simulink model "sample2"  (R2017b)
settings: Solver=VariableStepAuto  StartTime=0.0  StopTime=10.0  RelTol=1e-3
settings Model: Creator=aki  LastModifiedBy=aki

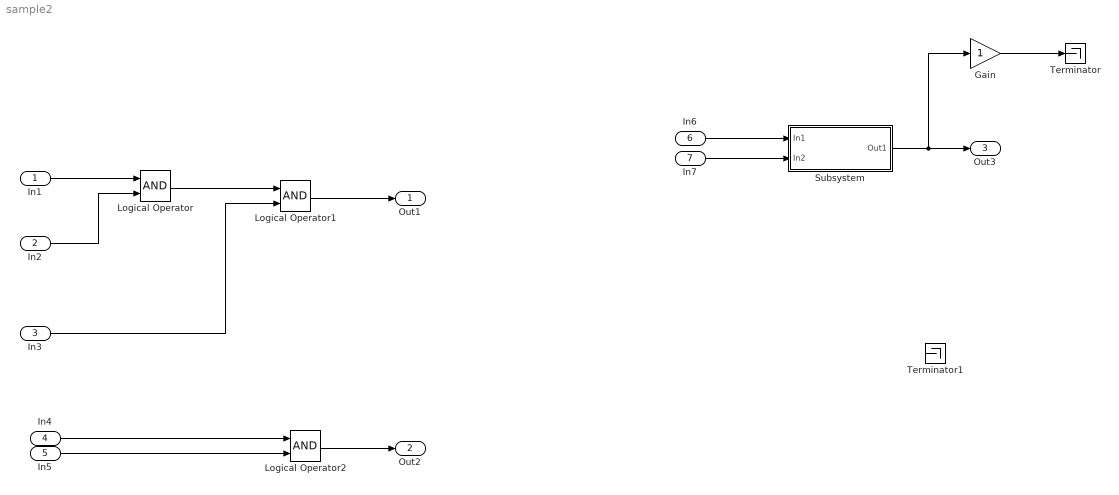
== system sample2 ==
  In1 : Inport
  In2 : Inport  Port=2
  In3 : Inport  Port=3
  In4 : Inport  Port=4
  In5 : Inport  Port=5
  In6 : Inport  Port=6
  In7 : Inport  Port=7
  Gain : Gain
  Logical Operator : Logic  AllPortsSameDT=off  OutDataTypeStr=boolean
  Logical Operator1 : Logic  AllPortsSameDT=off  OutDataTypeStr=boolean
  Logical Operator2 : Logic  AllPortsSameDT=off  OutDataTypeStr=boolean
  Subsystem : Subsystem
  Terminator : Terminator
  Terminator1 : Terminator
  Out1 : Outport
  Out2 : Outport  Port=2
  Out3 : Outport  Port=3
  wires:
  In1/1 -> Logical Operator/1
  In2/1 -> Logical Operator/2
  Logical Operator/1 -> Logical Operator1/1
  In3/1 -> Logical Operator1/2
  Logical Operator1/1 -> Out1/1
  In4/1 -> Logical Operator2/1
  In5/1 -> Logical Operator2/2
  Logical Operator2/1 -> Out2/1
  In6/1 -> Subsystem/1(In1)
  In7/1 -> Subsystem/2(In2)
  Subsystem/1(Out1) -> Gain/1, Out3/1
  Gain/1 -> Terminator/1

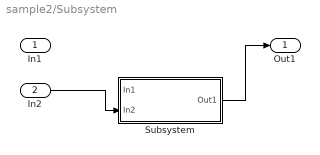
== system sample2/Subsystem ==
  In1 : Inport
  In2 : Inport  Port=2
  Subsystem : Subsystem
  Out1 : Outport
  wires:
  In2/1 -> Subsystem/2(In2)
  Subsystem/1(Out1) -> Out1/1

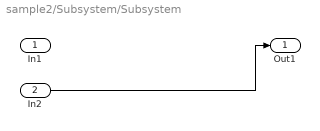
== system sample2/Subsystem/Subsystem ==
  In1 : Inport
  In2 : Inport  Port=2
  Out1 : Outport
  wires:
  In2/1 -> Out1/1
